simulink library "INT_EngDem_TrqLimCoord"  (R2016b)
settings: Solver=VariableStepAuto  StartTime=0.0  StopTime=10.0  RelTol=1e-3
settings Model: Creator=bianxuyin  LastModifiedBy=bianxuyin

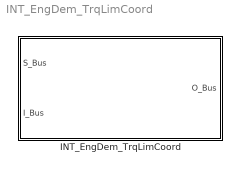
== system INT_EngDem_TrqLimCoord ==
  INT_EngDem_TrqLimCoord : Subsystem

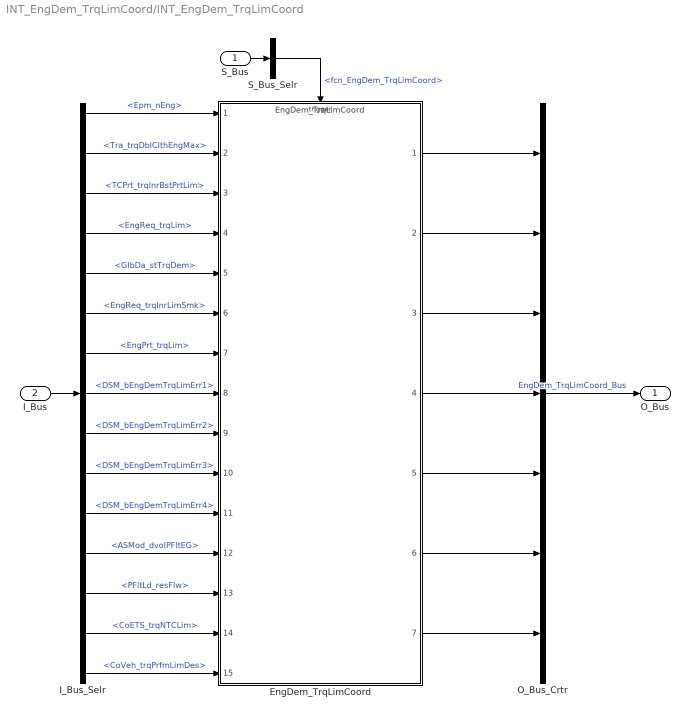
== system INT_EngDem_TrqLimCoord/INT_EngDem_TrqLimCoord ==
  S_Bus : Inport
  I_Bus : Inport  Port=2
  EngDem_TrqLimCoord : ModelReference  ModelNameDialog=EngDem_TrqLimCoord  SimulationMode=Normal  ModelReferenceVersion=1.59  TriggerPortName=function  TriggerPortTriggerType=function-call  TriggerPortStatesWhenEnabling=held
  I_Bus_Selr : BusSelector  OutputSignals=Epm_nEng,Tra_trqDblClthEngMax,TCPrt_trqInrBstPrtLim,EngReq_trqLim,GlbDa_stTrqDem,EngReq_trqInrLimSmk,EngPrt_trqLim,DSM_bEngDemTrqLimErr1,DSM_bEngDemTrqLimErr2,DSM_bEngDemTrqLimErr3,DSM_bEngDemTrqLimErr4,ASMod_dvolPFltEG,PFltLd_resFlw,CoETS_trqNTCLim,CoVeh_trqPrfmLimDes
  O_Bus_Crtr : BusCreator  Inputs=7
  S_Bus_Selr : BusSelector  OutputSignals=fcn_EngDem_TrqLimCoord
  O_Bus : Outport
  wires:
  S_Bus_Selr/1 -> EngDem_TrqLimCoord/Trigger  "<fcn_EngDem_TrqLimCoord>"
  S_Bus/1 -> S_Bus_Selr/1
  I_Bus/1 -> I_Bus_Selr/1
  I_Bus_Selr/1 -> EngDem_TrqLimCoord/1  "<Epm_nEng>"
  I_Bus_Selr/2 -> EngDem_TrqLimCoord/2  "<Tra_trqDblClthEngMax>"
  I_Bus_Selr/3 -> EngDem_TrqLimCoord/3  "<TCPrt_trqInrBstPrtLim>"
  I_Bus_Selr/4 -> EngDem_TrqLimCoord/4  "<EngReq_trqLim>"
  I_Bus_Selr/5 -> EngDem_TrqLimCoord/5  "<GlbDa_stTrqDem>"
  I_Bus_Selr/6 -> EngDem_TrqLimCoord/6  "<EngReq_trqInrLimSmk>"
  I_Bus_Selr/7 -> EngDem_TrqLimCoord/7  "<EngPrt_trqLim>"
  I_Bus_Selr/8 -> EngDem_TrqLimCoord/8  "<DSM_bEngDemTrqLimErr1>"
  I_Bus_Selr/9 -> EngDem_TrqLimCoord/9  "<DSM_bEngDemTrqLimErr2>"
  I_Bus_Selr/10 -> EngDem_TrqLimCoord/10  "<DSM_bEngDemTrqLimErr3>"
  I_Bus_Selr/11 -> EngDem_TrqLimCoord/11  "<DSM_bEngDemTrqLimErr4>"
  I_Bus_Selr/12 -> EngDem_TrqLimCoord/12  "<ASMod_dvolPFltEG>"
  I_Bus_Selr/13 -> EngDem_TrqLimCoord/13  "<PFltLd_resFlw>"
  I_Bus_Selr/14 -> EngDem_TrqLimCoord/14  "<CoETS_trqNTCLim>"
  I_Bus_Selr/15 -> EngDem_TrqLimCoord/15  "<CoVeh_trqPrfmLimDes>"
  O_Bus_Crtr/1 -> O_Bus/1  "EngDem_TrqLimCoord_Bus"
  EngDem_TrqLimCoord/1 -> O_Bus_Crtr/1
  EngDem_TrqLimCoord/2 -> O_Bus_Crtr/2
  EngDem_TrqLimCoord/3 -> O_Bus_Crtr/3
  EngDem_TrqLimCoord/4 -> O_Bus_Crtr/4
  EngDem_TrqLimCoord/5 -> O_Bus_Crtr/5
  EngDem_TrqLimCoord/6 -> O_Bus_Crtr/6
  EngDem_TrqLimCoord/7 -> O_Bus_Crtr/7
